simulink library "FDM_in"  (R2016b)
settings: Solver=VariableStepAuto  StartTime=0.0  StopTime=10.0  RelTol=1e-3
settings Model: Creator=mhussa27  LastModifiedBy=mhussa27

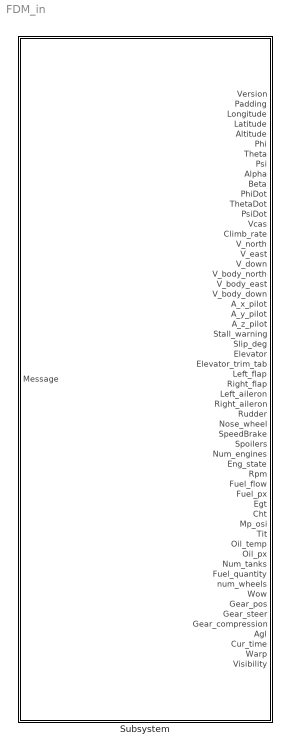
== system FDM_in ==
  Subsystem : Subsystem

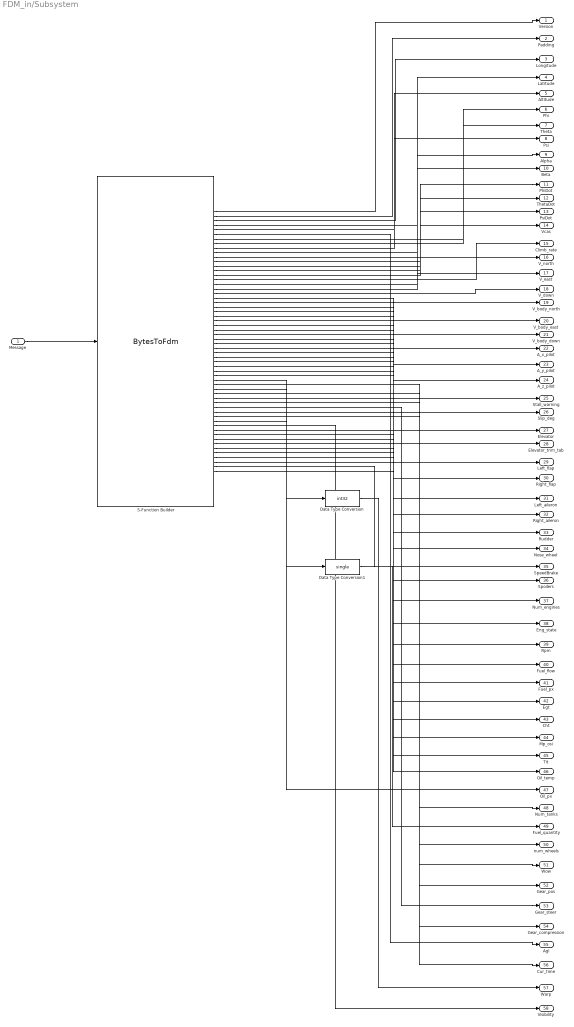
== system FDM_in/Subsystem ==
  Message : Inport
  Data Type Conversion : DataTypeConversion  OutDataTypeStr=int32
  Data Type Conversion1 : DataTypeConversion  OutDataTypeStr=single
  S-Function Builder : S-Function  InitFcn=try, set_param(gcb,'FunctionName','BytesToFdm'), end  FunctionName=BytesToFdm  SFunctionModules=BytesToFdm_wrapper  SFunctionDeploymentMode=off  EnableBusSupport=off  mask(S-Function Builder){}
      mask help: Simulink:masks:SFunctionBuilder_MD
      mask init:
      | val = [[.9  0.75 0.75 1 1 .9 .9 1]',[1 1 0.75 0.75 .9 .9 1 .9]'];try , sys = get_param(gcb,'SfunBuilderFcnName');if isempty(sys), sys = get_param(gcb,'FunctionName'); end,catch, sys = get_param(gcb,'FunctionName'); end
      settings: CopyFcn=set_param(gcbh,'LinkStatus','none')  PreSaveFcn=try, set_param(gcb,'FunctionName','BytesToFdm'), end  OpenFcn=sfunctionwizard(gcbh)
      mask Display:
      | plot(val(:,1),val(:,2))
      | disp(sys)
      | port_label('input',1,'Input')
      | port_label('output',1,'Version')
      | port_label('output',2,'padding')
      | port_label('output',3,'longitude')
      | port_label('output',4,'latitude')
      | port_label('output',5,'altitude')
      | port_label('output',6,'agl')
      | port_label('output',7,'phi')
      | port_label('output',8,'theta')
      | port_label('output',9,'psi')
      | port_label('output',10,'alpha')
      | port_label('output',11,'beta')
      | port_label('output',12,'phidot')
      | port_label('output',13,'thetadot')
      | port_label('output',14,'psidot')
      | port_label('output',15,'vcas')
      | port_label('output',16,'climb_rate')
      | port_label('output',17,'v_north')
      | port_label('output',18,'v_east')
      | port_label('output',19,'v_down')
      | port_label('output',20,'v_body_u')
      | port_label('output',21,'v_body_v')
      | port_label('output',22,'v_body_w')
      | port_label('output',23,'A_X_pilot')
      | port_label('output',24,'A_Y_pilot')
      | port_label('output',25,'A_Z_pilot')
      | port_label('output',26,'stall_warning')
      | port_label('output',27,'slip_deg')
      | port_label('output',28,'num_engines')
      | port_label('output',29,'eng_state')
      | port_label('output',30,'rpm')
      | port_label('output',31,'fuel_flow')
      | port_label('output',32,'fuel_px')
      | port_label('output',33,'egt')
      | port_label('output',34,'cht')
      | port_label('output',35,'mp_osi')
      | port_label('output',36,'tit')
      | port_label('output',37,'oil_temp')
      | port_label('output',38,'oil_px')
      | port_label('output',39,'num_tanks')
      | port_label('output',40,'fuel_quantity')
      | port_label('output',41,'num_wheels')
      | port_label('output',42,'wow')
      | port_label('output',43,'gear_pos')
      | port_label('output',44,'gear_steer')
      | port_label('output',45,'gear_compression')
      | port_label('output',46,'cur_time')
      | port_label('output',47,'warp')
      | port_label('output',48,'visibility')
      | port_label('output',49,'elevator')
      | port_label('output',50,'elevator_trim_tab')
      | port_label('output',51,'left_flap')
      | port_label('output',52,'right_flap')
      | port_label('output',53,'left_aileron')
      | port_label('output',54,'right_aileron')
      | port_label('output',55,'rudder')
      | port_label('output',56,'nose_wheel')
      | port_label('output',57,'speedbrake')
      | port_label('output',58,'spoilers')
  Version : Outport
  Padding : Outport  Port=2
  Longitude : Outport  Port=3
  Latitude : Outport  Port=4
  Altitude : Outport  Port=5
  Phi : Outport  Port=6
  Theta : Outport  Port=7
  Psi : Outport  Port=8
  Alpha : Outport  Port=9
  Beta : Outport  Port=10
  PhiDot : Outport  Port=11
  ThetaDot : Outport  Port=12
  PsiDot : Outport  Port=13
  Vcas : Outport  Port=14
  Climb_rate : Outport  Port=15
  V_north : Outport  Port=16
  V_east : Outport  Port=17
  V_down : Outport  Port=18
  V_body_north : Outport  Port=19
  V_body_east : Outport  Port=20
  V_body_down : Outport  Port=21
  A_x_pilot : Outport  Port=22
  A_y_pilot : Outport  Port=23
  A_z_pilot : Outport  Port=24
  Stall_warning : Outport  Port=25
  Slip_deg : Outport  Port=26
  Elevator : Outport  Port=27
  Elevator_trim_tab : Outport  Port=28
  Left_flap : Outport  Port=29
  Right_flap : Outport  Port=30
  Left_aileron : Outport  Port=31
  Right_aileron : Outport  Port=32
  Rudder : Outport  Port=33
  Nose_wheel : Outport  Port=34
  SpeedBrake : Outport  Port=35
  Spoilers : Outport  Port=36
  Num_engines : Outport  Port=37
  Eng_state : Outport  Port=38
  Rpm : Outport  Port=39
  Fuel_flow : Outport  Port=40
  Fuel_px : Outport  Port=41
  Egt : Outport  Port=42
  Cht : Outport  Port=43
  Mp_osi : Outport  Port=44
  Tit : Outport  Port=45
  Oil_temp : Outport  Port=46
  Oil_px : Outport  Port=47
  Num_tanks : Outport  Port=48
  Fuel_quantity : Outport  Port=49
  num_wheels : Outport  Port=50
  Wow : Outport  Port=51
  Gear_pos : Outport  Port=52
  Gear_steer : Outport  Port=53
  Gear_compression : Outport  Port=54
  Agl : Outport  Port=55
  Cur_time : Outport  Port=56
  Warp : Outport  Port=57
  Visibility : Outport  Port=58
  wires:
  S-Function Builder/2 -> Padding/1
  S-Function Builder/1 -> Version/1
  S-Function Builder/5 -> Altitude/1
  S-Function Builder/4 -> Latitude/1
  S-Function Builder/12 -> PhiDot/1
  S-Function Builder/11 -> Beta/1
  S-Function Builder/3 -> Longitude/1
  S-Function Builder/10 -> Alpha/1
  S-Function Builder/41 -> num_wheels/1
  S-Function Builder/48 -> Visibility/1
  S-Function Builder/46 -> Cur_time/1
  S-Function Builder/36 -> Tit/1
  S-Function Builder/33 -> Egt/1
  S-Function Builder/42 -> Wow/1
  S-Function Builder/6 -> Agl/1
  S-Function Builder/44 -> Gear_steer/1
  S-Function Builder/34 -> Cht/1
  S-Function Builder/32 -> Fuel_px/1
  S-Function Builder/38 -> Oil_px/1
  S-Function Builder/43 -> Gear_pos/1
  Data Type Conversion1/1 -> Fuel_quantity/1
  S-Function Builder/45 -> Gear_compression/1
  S-Function Builder/35 -> Mp_osi/1
  S-Function Builder/39 -> Num_tanks/1
  Data Type Conversion/1 -> Warp/1
  S-Function Builder/37 -> Oil_temp/1
  S-Function Builder/40 -> Data Type Conversion1/1
  S-Function Builder/47 -> Data Type Conversion/1
  S-Function Builder/26 -> Stall_warning/1
  S-Function Builder/25 -> A_z_pilot/1
  S-Function Builder/22 -> V_body_down/1
  S-Function Builder/8 -> Theta/1
  S-Function Builder/57 -> SpeedBrake/1
  S-Function Builder/30 -> Rpm/1
  S-Function Builder/21 -> V_body_east/1
  S-Function Builder/51 -> Left_flap/1
  S-Function Builder/54 -> Right_aileron/1
  S-Function Builder/31 -> Fuel_flow/1
  S-Function Builder/50 -> Elevator_trim_tab/1
  S-Function Builder/19 -> V_down/1
  S-Function Builder/53 -> Left_aileron/1
  S-Function Builder/29 -> Eng_state/1
  S-Function Builder/20 -> V_body_north/1
  S-Function Builder/28 -> Num_engines/1
  S-Function Builder/58 -> Spoilers/1
  S-Function Builder/13 -> ThetaDot/1
  S-Function Builder/17 -> V_north/1
  S-Function Builder/56 -> Nose_wheel/1
  S-Function Builder/55 -> Rudder/1
  S-Function Builder/52 -> Right_flap/1
  S-Function Builder/15 -> Vcas/1
  S-Function Builder/24 -> A_y_pilot/1
  S-Function Builder/27 -> Slip_deg/1
  S-Function Builder/23 -> A_x_pilot/1
  S-Function Builder/7 -> Phi/1
  S-Function Builder/18 -> V_east/1
  S-Function Builder/9 -> Psi/1
  S-Function Builder/49 -> Elevator/1
  S-Function Builder/14 -> PsiDot/1
  S-Function Builder/16 -> Climb_rate/1
  Message/1 -> S-Function Builder/1
